simulink model "udpTest"  (R2021b)
settings: Solver=VariableStepAuto  StartTime=0.0  StopTime=inf  RelTol=1e-3
libraries: dspnetwork x2, simulink x1, dspvision x1
settings Model: PacingRate=0.500000  Creator=GH  LastModifiedBy=GH

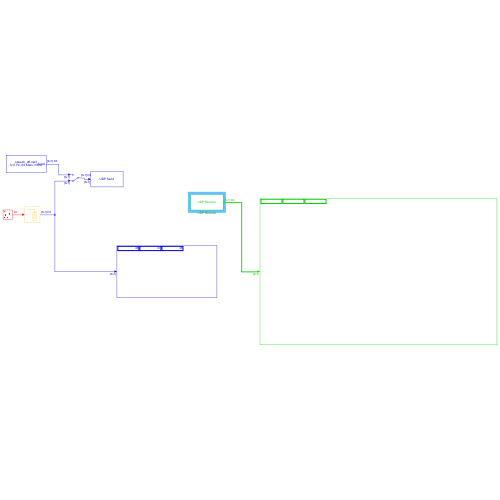
[thumbnail: Simulink's stored preview of the top-level diagram]
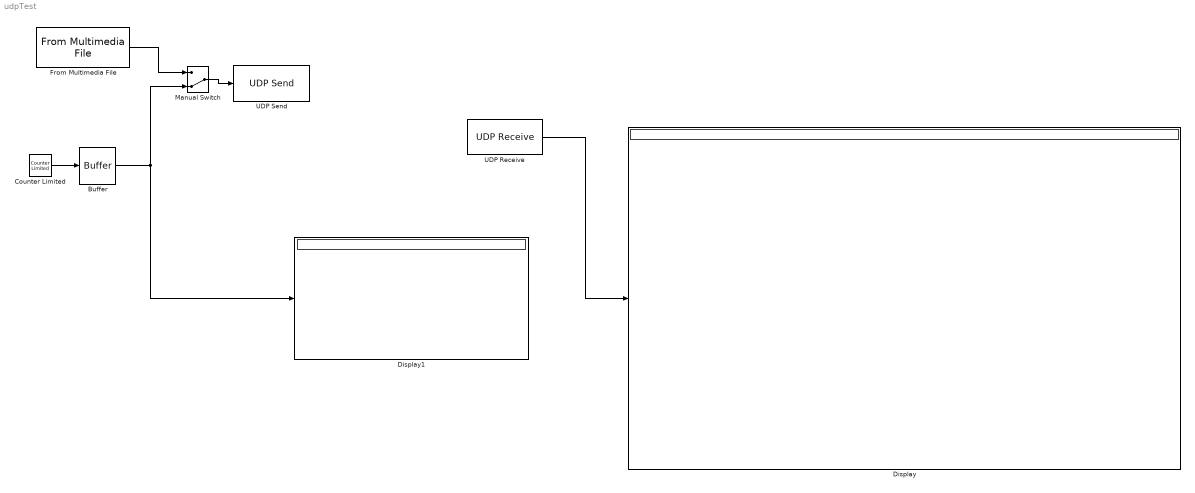
== system udpTest ==
  Buffer : Buffer  N=3  OutputFrames=off
  Counter Limited : simulink/Sources/Counter Limited  uplimit=999  tsamp=0.5/3
  Display : Display
  Display1 : Display
  From Multimedia File : dspvision/From Multimedia File  inputFilename=speech_dft.mp3  readRange=[1 Inf]  loop=on  numPlays=inf  outputStreams=Audio only  videoDataType=single  audioDataType=double  inheritSampleTime=off  userDefinedSampleTime=1/2  noAudioOutput=off  isIntensityVideo=off  fourcc=RGB  colorVideoFormat=Separate color signals  outputEOF=off  dataOrg=Column-major  audioFrameSize=3  computeAudioFrameSize=off  outSamplingMode=Sample based
  Manual Switch : ManualSwitch  CurrentSetting=0
  UDP Receive : dspnetwork/UDP Receive  localURL='0.0.0.0'  localPort=25000  remoteURL='0.0.0.0'  remotePort=-1  recvBufferSize=100  dims=3  signalDatatype=double  isComplex=off  isVarSize=on  showBlockingTime=off  blockingTime=0  sampletime=0.25  blockPlatform=[]
  UDP Send : dspnetwork/UDP Send  remoteURL='127.0.0.1'  remotePort=25000  localURL='0.0.0.0'  localPortSource=Automatically determine  localPort=-1  sendBufferSize=8192  sampletime=-1  blockPlatform=[]  separateLengthPort=0
  wires:
  UDP Receive/1 -> Display/1
  Manual Switch/1 -> UDP Send/1
  From Multimedia File/1 -> Manual Switch/1
  Counter Limited/1 -> Buffer/1
  Buffer/1 -> Display1/1, Manual Switch/2
